simulink model "suspensionSystem"  (R2020a)
settings: Solver=VariableStepAuto  StartTime=0.0  StopTime=50.0  MaxStep=0.001  RelTol=1e-3
undefined symbols (not defined in the file): Cs, Ks, Kt, MS, Mu, sigbuilder_block
settings Model: Creator=Admin  LastModifiedBy=Admin

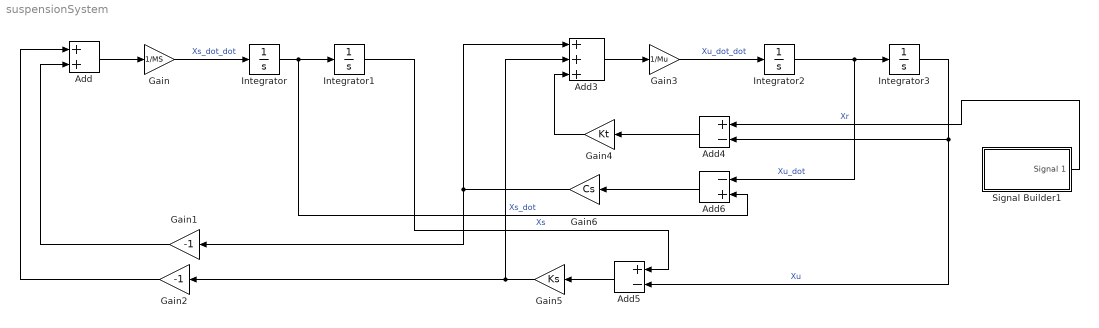
== system suspensionSystem ==
  Add : Sum
  Add3 : Sum  Inputs=+++
  Add4 : Sum  Inputs=+-
  Add5 : Sum  Inputs=+-
  Add6 : Sum  Inputs=-+
  Gain : Gain  Gain=1/MS
  Gain1 : Gain  Gain=-1
  Gain2 : Gain  Gain=-1
  Gain3 : Gain  Gain=1/Mu
  Gain4 : Gain  Gain=Kt
  Gain5 : Gain  Gain=Ks
  Gain6 : Gain  Gain=Cs
  Integrator{,1..3} (4 alike) : Integrator
  Signal Builder1 : Subsystem  Tag=STV Subsys  LoadFcn=sigbuilder_block('load');  StartFcn=sigbuilder_block('start');  StopFcn=sigbuilder_block('stop');  ClipboardFcn=sigbuilder_block('clipboard');  mask(Sigbuilder block){tuvar=[0:10]}
      mask help: Simulink:masks:SigbuilderBlock_MD
      mask init:
      | if ~strcmp(get_param(bdroot(gcbh),'SimulationStatus'),'stopped') tuvar = sigbuilder_block('maskInit'); end
      settings: CopyFcn=sigbuilder_block('copy');  DeleteFcn=sigbuilder_block('delete');  ModelCloseFcn=sigbuilder_block('modelClose');  PreSaveFcn=sigbuilder_block('preSave');  PauseFcn=sigbuilder_block('pause');  ContinueFcn=sigbuilder_block('continue');  NameChangeFcn=sigbuilder_block('namechange');  OpenFcn=sigbuilder_block('open',[437.6 199.2 550.4 400 ]);  CloseFcn=sigbuilder_block('close');
      mask Display: plot(0, 0, 100, 100,[2, 2, 32, 32, 2], [68, 8, 8, 68, 68],[32, 2], [38, 38], [32, 19, 2],[53, 60, 44], [32, 17, 17, 2],[16, 16, 31, 31]);txt = getActiveGroup(gcbh);text(2, 100, txt,'verticalAlignment', 'top');
  wires:
  Gain/1 -> Integrator/1  "Xs_dot_dot"
  Integrator/1 -> Integrator1/1, Add6/2  "Xs_dot"
  Integrator1/1 -> Add5/1  "Xs"
  Add/1 -> Gain/1
  Gain1/1 -> Add/2
  Gain2/1 -> Add/1
  Gain3/1 -> Integrator2/1  "Xu_dot_dot"
  Integrator2/1 -> Add6/1, Integrator3/1  "Xu_dot"
  Integrator3/1 -> Add4/2, Add5/2  "Xu"
  Add3/1 -> Gain3/1
  Add4/1 -> Gain4/1
  Add5/1 -> Gain5/1
  Signal Builder1/1(Signal 1) -> Add4/1  "Xr"
  Gain5/1 -> Add3/2, Gain2/1
  Gain6/1 -> Add3/1, Gain1/1
  Add6/1 -> Gain6/1
  Gain4/1 -> Add3/3

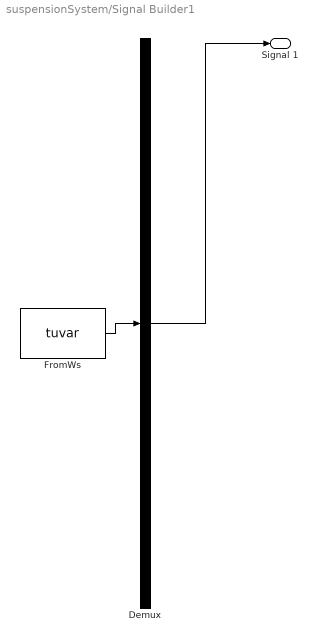
== system suspensionSystem/Signal Builder1 ==
  Demux : Demux  Tag=STV Demux  Outputs=1
      settings: DisplayOption=none
  FromWs : FromWorkspace  Tag=STV FromWs  VariableName=tuvar
      SigBuilderData=|
      | common.afterFinalStr = 'Extrapolate'
      | common.sampleTime = 0
      | dataSet.timeRange = [0 50]
      | dataSet.name = 'Group 1'
      | sbobj.Groups.Name = 'Group 1'
      | sbobj.Groups.Signals.Name = 'Signal 1'
      | sbobj.Groups.Signals.XData = [0 0.5 1 1 1.5 2 2 2.5 2.5 3 3 3.5 4 4.5 4.5 5 5 5.5 5.5 6 6 6.5 6.5 7 7 7.5 7.5 8 8 8.5 8.5 9 9 9.5 10 10 10.5 10.5 11 11 11.5 11.5 12 12 12.5 12.5 13 13 13.5 13.5 14 14 14.5 14.5 15 15 15.5 15.5 16 16 16.5 16.5 17 17 17.5 17.5 18 18 18.5 18.5 19 19 19.5 19.5 20 20 20.5 20.5 21 21 21.5 21.5 22 22 22.5 22.5 23 23 23.5 23.5 24 24 24.5 24.5 25 25 25.5 25.5 26 26 26.5 26.5 27 27 27.5 27.5 28 28 28.5 28.5 29 29 29.5 29.5 30 30 30.5 30.5 31 31 31.5 31.5 32 32 32.5 32.5 33 33 33.5 33.5 34 34 34.5 34.5 35 35 35.5 35.5 36 36 36.5 36.5 37 37 37.5 37.5 38 38 38.5 38.5 39 39 39.5 39.5 40 40 40.5 40.5 41 41 41.5 41.5 42 42 42.5 42.5 43 43 43.5 43.5 44 44 44.5 44.5 45 45 45.5 45.5 46 46 46.5 46.5 47 47 47.5 47.5 48 48 48.5 48.5 49 49 49.5 49.5 50]
      | sbobj.Groups.Signals.YData = [-0.01 -0.01 -0.01 1.99 2.01 2.01 2 2 2.01 2.01 2 2 2 2 0 0 1.03 1.58 1.59 1.6 2 2 0 0 2 2 0 0 2 2 -0.33 -0.32 -0.3 -0.32 -0.3 -0.32 -0.28 0 0 2 2 0 0 2 2 0 0 2 2 0 0 2 2 0 0 2 2 0 0 2 2 0 0 2 2 0 0 2 2 0 0 2 2 0 0 2 2 0 0 2 2 1.97 1.43 1.11 2 0 0 2 2 0 0 2 2 0 0 2 2 0 0 2 2 0 0 2 2 0 0 2 2 0 0 2 2 0 0 2 2 0 0 2 2 0 0 2 2 0 0 2 2 0 0 2 2 0 0 2 2 0 0 -0.01 2 0 0 2 2 0 0 2 2 0 0 2 2 0 0 2 2 0 0 2 2 0 0 2 2 0 0 2 2 0 0 2 2 0 0 2 2 0 0 2 2 0 0 2 2 0 0 2 2 0 0 2 2 0 0]
      | sbobj.Groups.TimeRange = [0 50]
  Signal 1 : Outport  Tag=STV Outport
  wires:
  FromWs/1 -> Demux/1
  Demux/1 -> Signal 1/1
